simulink model "hyd_hyb_2_fuz"  (Simulink 7.7)
settings: Solver=ode14x  StartTime=0  StopTime=1089  FixedStep=0.01  MaxStep=.4  RelTol=1e-8
InitFcn:
  | const_3
values from neighbouring files (symbols this model uses):
  Af = 6.3    [brk_enrg.m]    (also in brk_enrg_1.m)
  BSFC_906_205 = [3.5684 4.3466 5.1668 6.0769 6.988 7.8992 8.8104 9.7336 10.8548 11.9809 13.1112 14.2571 ... (663 elements, 39x17)]    [BSFC_map_906_205.mat]
  Cd = 0.55    [brk_enrg.m]    (also in brk_enrg_1.m)
  den = 1.202    [brk_enrg.m]    (also in brk_enrg_1.m)
  fr = 0.01    [brk_enrg.m]    (also in brk_enrg_1.m)
undefined symbols (not defined in the file or in its folder): clutchRise, down_spd_2, down_spd_3, down_spd_4, down_spd_c, fuel_density, gearshift, I_wheel, Idle_spd_eng_906, M1_hydr, p_v_15, pmax_125, qv_125, Rw, sec_eng_sfc_map, T_max_906, T_min, TC_spd_ratio_max, torque_convertor, Twait, up_spd_1, up_spd_2, up_spd_3, up_spd_c, v_p_10, v_p_15, v_p_5
libraries: fl_lib x43, nesl_utility x30, sdl_lib x14, simulink x4, fuzblock x1, simulink_need_slupdate x1
(part 3 of 3)

== system hyd_hyb_2_fuz/Transmission1/Torque Convertor/main solver/Sensor(TC_out)/Motion sensor ==
  Ideal Rotational Motion Sensor : fl_lib/Mechanical/Mechanical Sensors/Ideal Rotational Motion Sensor  SystemSampleTime=-1  offset=0 rad  w_Log=off  t_Log=off  phi_Log=off  LocalVarNames=|w|t|phi  LocalVarDescs=|w|t|phi  LocalVarLogging=[]
  MRR : fl_lib/Mechanical/Rotational Elements/Mechanical Rotational Reference  SystemSampleTime=-1  t_Log=off  LocalVarNames=|t  LocalVarDescs=|t  LocalVarLogging=[]
  PS-Simulink Converter : nesl_utility/PS-Simulink Converter  SystemSampleTime=-1  PhysicalDomain=network_engine_domain  LeftPortType=input  RightPortType=output  SubClassName=ps_output  Unit=rad/s  AffineConversion=off
  A : PMIOPort  Port=1  Side=Left
  W : Outport
  wires:
  PS-Simulink Converter/1 -> W/1
  connections:
  MRR/LConn1 -- Ideal Rotational Motion Sensor/RConn1
  Ideal Rotational Motion Sensor/RConn2 -- PS-Simulink Converter/LConn1
  A/RConn1 -- Ideal Rotational Motion Sensor/LConn1

== system hyd_hyb_2_fuz/Transmission1/Torque Convertor/main solver/Sensor(TC_out)/Torque sensor ==
  PS2S : nesl_utility/PS-Simulink Converter  SystemSampleTime=-1  PhysicalDomain=network_engine_domain  LeftPortType=input  RightPortType=output  SubClassName=ps_output  Unit=1  AffineConversion=off
  Torque Sensor : fl_lib/Mechanical/Mechanical Sensors/Ideal Torque Sensor  SystemSampleTime=-1  w_Log=off  t_Log=off  LocalVarNames=|w|t  LocalVarDescs=|w|t  LocalVarLogging=[]
  B : PMIOPort  Port=1  Side=Right
  A : PMIOPort  Port=2  Side=Left
  T : Outport
  wires:
  PS2S/1 -> T/1
  connections:
  Torque Sensor/RConn2 -- PS2S/LConn1
  B/RConn1 -- Torque Sensor/RConn1
  A/RConn1 -- Torque Sensor/LConn1

== system hyd_hyb_2_fuz/Transmission1/gear box/gear box/Clutch Control/Enabled Subsystem1 ==
  Enable : EnablePort  StatesWhenEnabling=reset  PropagateVarSize=During execution
  Clutch A Actuator : TransferFcn  Numerator=[1/clutchRise]  Denominator=[1 1/clutchRise]
  engage : Constant
  clutch release : Outport  OutputWhenDisabled=reset  InitialOutput=[0]
  wires:
  engage/1 -> Clutch A Actuator/1
  Clutch A Actuator/1 -> clutch release/1

== system hyd_hyb_2_fuz/Transmission1/gear box/gear box/Clutch Control/Enabled Subsystem2 ==
  Enable : EnablePort  StatesWhenEnabling=reset  PropagateVarSize=During execution
  Clutch A Actuator : TransferFcn  Numerator=[1/clutchRise]  Denominator=[1 1/clutchRise]
  engage : Constant
  clutch release : Outport  OutputWhenDisabled=reset  InitialOutput=[0]
  wires:
  Clutch A Actuator/1 -> clutch release/1
  engage/1 -> Clutch A Actuator/1

== system hyd_hyb_2_fuz/Transmission1/gear box/gear box/Clutch Control/Enabled Subsystem3 ==
  Enable : EnablePort  StatesWhenEnabling=reset  PropagateVarSize=During execution
  Clutch A Actuator : TransferFcn  Numerator=[1/clutchRise]  Denominator=[1 1/clutchRise]
  engage : Constant
  clutch release : Outport  OutputWhenDisabled=reset  InitialOutput=[0]
  wires:
  engage/1 -> Clutch A Actuator/1
  Clutch A Actuator/1 -> clutch release/1

== system hyd_hyb_2_fuz/Transmission1/gear box/gear box/Clutch Control/Enabled Subsystem4 ==
  Enable : EnablePort  StatesWhenEnabling=reset  PropagateVarSize=During execution
  Clutch A Actuator : TransferFcn  Numerator=[1/clutchRise]  Denominator=[1 1/clutchRise]
  engage : Constant
  clutch release : Outport  OutputWhenDisabled=reset  InitialOutput=[0]
  wires:
  Clutch A Actuator/1 -> clutch release/1
  engage/1 -> Clutch A Actuator/1

== stateflow chart driver/Chart ==
  state transmission state control [group]
    state Drive
      during: s=1;
    state Neutral
      during: s=0;
    (default) -> Neutral
    Neutral -> Drive : [cyc> 0]
    Drive -> Neutral : after(1,sec)[cyc== 0]
  data: cyc input double; speed input double; s output double

== stateflow chart Transmission1/transmission control/Chart1 ==
  state fourth
    entry: gear = 4;
  state third
    entry: gear = 3;
  state second
    entry: gear = 2;
  state first
    entry: TC=1;
  state firstc
    entry: gear=1;
    entry: TC=0;
  second -> third [order 1] : after(Twait,tick)
      | [speed >= up_spd_2]
  first -> second [order 1] : after(Twait,tick)
      | [speed >= up_spd_1]
  third -> fourth [order 1] : after(Twait,tick)
      | [speed >= up_spd_3]
  firstc -> first : after(Twait,tick)
      | [speed >=up_spd_c]
  (default) -> firstc
  third -> second [order 2] : after(Twait,tick)
      | [speed < down_spd_3]
  fourth -> third : after(Twait,tick)
      | [speed < down_spd_4]
  first -> firstc [order 2] : after(Twait,tick)
      | [speed < down_spd_c]
  second -> first [order 2] : after(Twait,tick)
      | [speed < down_spd_2]
  data: speed input double; gear output double; TC output double; down_spd_4 parameter double; down_spd_2 parameter double; down_spd_3 parameter double; up_spd_1 parameter double; up_spd_2 parameter double; up_spd_3 parameter double; down_spd_c parameter double; up_spd_c parameter double; Twait parameter double

== matlab function controller/MATLAB Function ==
  data: T_pm input double; T_eng output double; T_brk input double; T_mech_brk output double; T_dem input double
function [T_eng,T_mech_brk] = fcn(T_pm,T_brk,T_dem)
if abs(T_brk)>0.1
    T_eng=0;
    T_mech_brk=min(0,T_brk-T_pm);
else    
    T_mech_brk=0;
    T_eng=max(0,T_dem-T_pm);
end
end

== stateflow chart hydraulic transmission/PM_hydraulic_machine /qv - pmax evaluation/Chart ==
  state state1
    during: u1=1;
  state state2
    during: u1=0;
  (default) -> state1
  state1 -> state2 : [soc <= soc_min]
  state2 -> state1 : [soc > 50]
  data: soc input double; soc_min input double; u1 output double
